simulink model "Podstawowe_modele"  (R2024b)
settings: Solver=ode4  StartTime=0.0  StopTime=10.0  FixedStep=0.01  RelTol=1e-3
settings Model: Creator=mati  LastModifiedBy=mati

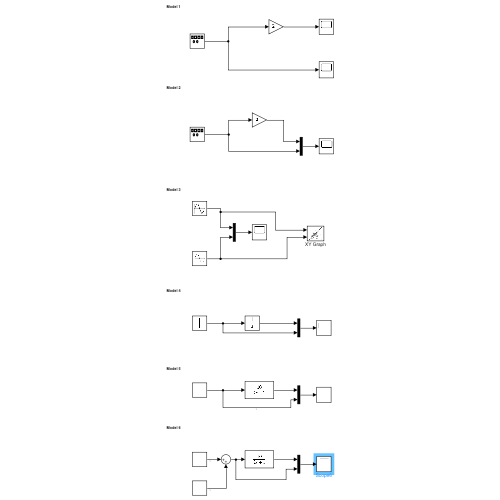
[thumbnail: Simulink's stored preview of the top-level diagram]
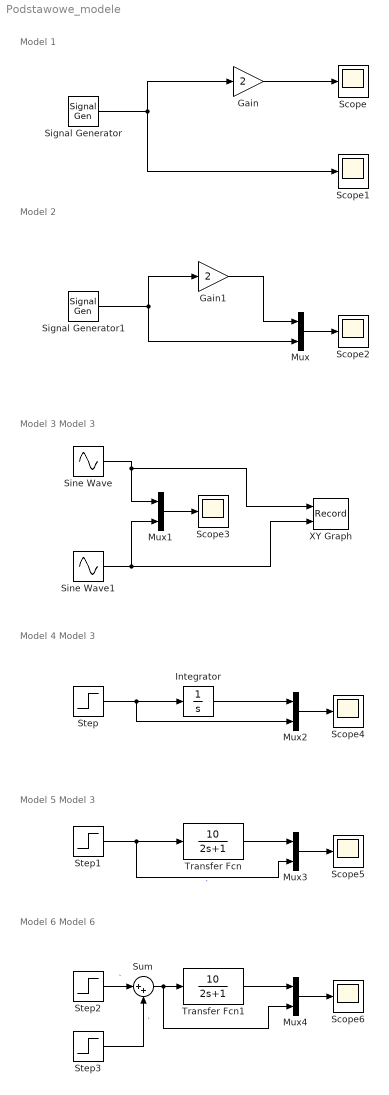
== system Podstawowe_modele ==
  note: Model 1
  note: Model 2
  note: Model 3
      | Model 3
  note: Model 5
      | Model 3
  note: Model 6
      | Model 6
  note: Model 4
      | Model 3
  Gain : Gain  Gain=2
  Gain1 : Gain  Gain=2
  Integrator : Integrator
  Mux{,1..4} (5 alike) : Mux  Inputs=2
  Scope{,1..6} (7 alike) : Scope
  Signal Generator : SignalGenerator  Units=rad/sec
  Signal Generator1 : SignalGenerator  Units=rad/sec
  Sine Wave : Sin  Amplitude=2  Frequency=3  SampleTime=0
  Sine Wave1 : Sin  Frequency=2  SampleTime=0
  Step : Step  SampleTime=0
  Step1 : Step  SampleTime=0
  Step2 : Step  Time=0  After=10  SampleTime=0
  Step3 : Step  Time=0.1  After=-10  SampleTime=0
  Sum : Sum  Inputs=|++
  Transfer Fcn : TransferFcn  Numerator=10  Denominator=[2 1]
  Transfer Fcn1 : TransferFcn  Numerator=10  Denominator=[2 1]
  XY Graph : Record  FileSettingsInternal="{\"entries\":[{\"content\":{\"excelSettings\":{\"content\":{},\"type\":\"Streamout.ExcelSettings\"}},\"type\":\"Streamout.FileSettingStorage\",\"uuid\":\"\"}],\"packageUris\":[\"http:\\/\\/schema.mathworks.com\\/mf0\\/streamout_blocks\\/R2020a\"],\"version\":\"1.0\"}"  Layout=[1 1]  SignalsInternal="{\"entries\":[{\"content\":{\"signals\":[{\"content\":{\"blockPath\":[],\"dimensions\":[1],\"domain\":\"\",\"lineColor\":\"#a2142f\",\"plots\":[ 1 ],\"port\":1,\"sid\":[\"\"],\"signalID\":1,\"signalName\":\"Sine Wave\"},\"type\":\"RecordBlkView.Signal\",\"uuid\":\"\"},{\"content\":{\"blockPath\":[],\"dimensions\":[1],\"domain\":\"\",\"lineColor\":\"#139fff\",\"plots\":[ 1 ],\"port\":2,\"sid\":[\"\"],\"signalID\":2,\"signalName\":\"Sine Wave1\"},\"type\":\"RecordBlkView.Signal\",\"uuid\":\"\"}]},\"type\":\"RecordBlkView.InputSignals\",\"uuid\":\"\"}],\"packageUris\":[\"http:\\/\\/schema.mathworks.com\\/mf0\\/streamout_blocks\\/R2020a\"],\"version\":\"1.0\"}"  VisualizationBindings="{\"xyplotplugin\":{\"info\":[{\"series\":[{\"bindingParametersList\":[{\"parameter\":\"X-Axis\",\"signalID\":1,\"signalName\":\"Sine Wave\"},{\"parameter\":\"Y-Axis\",\"signalID\":2,\"signalName\":\"Sine Wave1\"}],\"seriesID\":0}],\"subplotID\":1}]}}"  CompatibilityTag=XY
  wires:
  Signal Generator/1 -> Scope1/1, Gain/1
  Gain/1 -> Scope/1
  Signal Generator1/1 -> Gain1/1, Mux/2
  Mux/1 -> Scope2/1
  Gain1/1 -> Mux/1
  Mux1/1 -> Scope3/1
  Sine Wave/1 -> XY Graph/1, Mux1/1
  Sine Wave1/1 -> XY Graph/2, Mux1/2
  Step/1 -> Mux2/2, Integrator/1
  Mux2/1 -> Scope4/1
  Integrator/1 -> Mux2/1
  Step1/1 -> Transfer Fcn/1, Mux3/2  "`"
  Mux3/1 -> Scope5/1
  Transfer Fcn/1 -> Mux3/1
  Mux4/1 -> Scope6/1
  Transfer Fcn1/1 -> Mux4/1
  Step2/1 -> Sum/1  "`"
  Sum/1 -> Mux4/2, Transfer Fcn1/1
  Step3/1 -> Sum/2  "`"
